simulink model "lab3"  (R2022b)
settings: Solver=FixedStepAuto  StartTime=0.0  StopTime=300  FixedStep=0.05  RelTol=1e-3
undefined symbols (not defined in the file): g, k, m
settings Model: Creator=dambi  LastModifiedBy=dambi

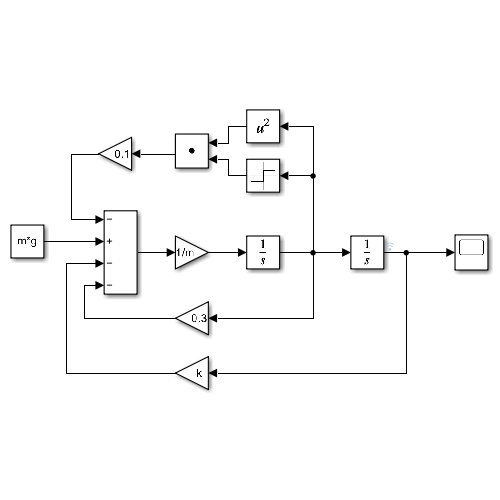
[thumbnail: Simulink's stored preview of the top-level diagram]
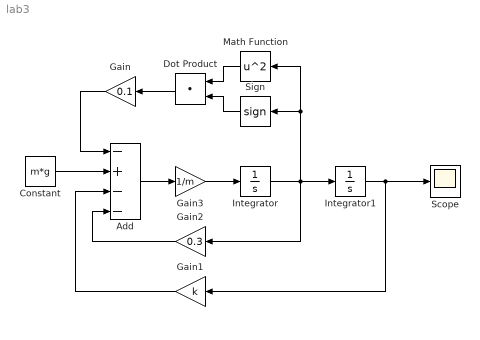
== system lab3 ==
  Add : Sum  Inputs=-+--
  Constant : Constant  Value=m*g
  Dot Product : DotProduct  OutDataTypeStr=Inherit: Inherit via internal rule
  Gain : Gain  Gain=0.1
  Gain1 : Gain  Gain=k
  Gain2 : Gain  Gain=0.3
  Gain3 : Gain  Gain=1/m
  Integrator : Integrator
  Integrator1 : Integrator
  Math Function : Math  Operator=square
  Scope : Scope
  Sign : Signum
  wires:
  Constant/1 -> Add/2
  Gain/1 -> Add/1
  Gain2/1 -> Add/4
  Gain1/1 -> Add/3
  Add/1 -> Gain3/1
  Gain3/1 -> Integrator/1
  Dot Product/1 -> Gain/1
  Sign/1 -> Dot Product/2
  Math Function/1 -> Dot Product/1
  Integrator/1 -> Integrator1/1, Gain2/1, Math Function/1, Sign/1
  Integrator1/1 -> Scope/1, Gain1/1
